simulink model "exam3"  (R2022b)
settings: Solver=VariableStepAuto  StartTime=0.0  StopTime=10.0  RelTol=1e-3
settings Model: Creator=devak  LastModifiedBy=devak

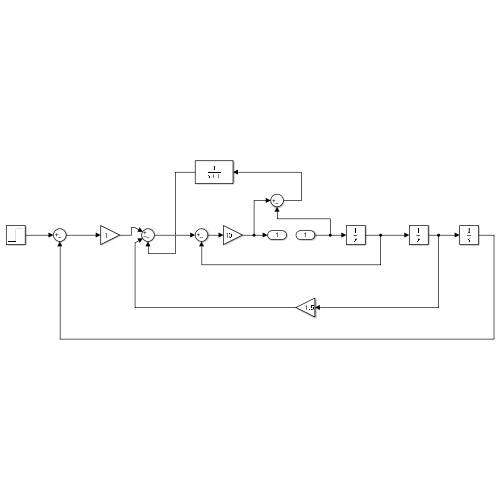
[thumbnail: Simulink's stored preview of the top-level diagram]
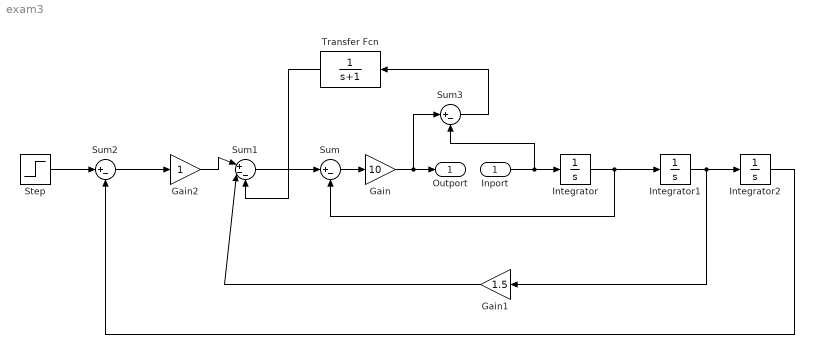
== system exam3 ==
  Inport : Inport
  Gain : Gain  Gain=10
  Gain1 : Gain  Gain=1.5
  Gain2 : Gain
  Integrator : Integrator
  Integrator1 : Integrator
  Integrator2 : Integrator
  Step : Step  After=1.50615  SampleTime=0
  Sum : Sum  Inputs=|+-
  Sum1 : Sum  Inputs=|+--
  Sum2 : Sum  Inputs=|+-
  Sum3 : Sum  Inputs=|+-
  Transfer Fcn : TransferFcn  Denominator=[1 1]
  Outport : Outport
  wires:
  Inport/1 -> Sum3/2, Integrator/1
  Gain/1 -> Sum3/1, Outport/1
  Sum1/1 -> Sum/1
  Gain2/1 -> Sum1/1
  Step/1 -> Sum2/1
  Sum2/1 -> Gain2/1
  Integrator1/1 -> Gain1/1, Integrator2/1
  Sum/1 -> Gain/1
  Sum3/1 -> Transfer Fcn/1
  Integrator2/1 -> Sum2/2
  Transfer Fcn/1 -> Sum1/3
  Integrator/1 -> Integrator1/1, Sum/2
  Gain1/1 -> Sum1/2
